simulink model "CtrlEdosObs0x2810x29"  (R2023a)
settings: Solver=ode4  StartTime=0.0  StopTime=5  FixedStep=0.001  RelTol=1e-3
values from neighbouring files (symbols this model uses):
  A = [-6 -3 -2;22 5 10;-12 0 -7]    [eje4_par3.m]    (also in ejer1_par3.m = [9 -28 -40; 10 -28 -35;-4 11 12]; ejer2_par3.m = [8 -12 4;3 -4 1;-21 30 -11]; ejer3_par3.m = [101 -6 56;-121 4 -65;-208 12 -115]; ejer5_par3.m = [-16 -25 25; -7 -12 9;-17 -26 23])
  B = [-8;11;9]    [eje4_par3.m]    (also in ejer2_par3.m = [6;-6;-32]; ejer3_par3.m = [-1;2;2]; ejer5_par3.m = [-2;0;-2])
  C = [50 20 22]    [eje4_par3.m]    (also in ejer3_par3.m = [-108 6 -58])
  k = place(A,B,lamC)    [eje4_par3.m]    (also in ejer5_par3.m = inv(R)*B'*Pk)
  L = place(A',C',lamObs')'    [eje4_par3.m]    (also in ejer3_par3.m = place(A',C',lamR')')
  Ueq1 = 3    [eje4_par3.m]    (also in ejer2_par3.m = 10)
  x0 = [3;-9;8]    [eje4_par3.m]    (also in ejer2_par3.m = [-3,9,-10]; ejer3_par3.m = [-10;-7;-7])
  x0h = [0;0;0]    [eje4_par3.m]    (also in ejer3_par3.m)
  Xeq1 = mldivide(Aeq,-Beq)    [eje4_par3.m]    (also in ejer2_par3.m)
settings Model: Creator=itzel  LastModifiedBy=userh
settings OptimizationCC: ReuseModelBlockBuffer=off

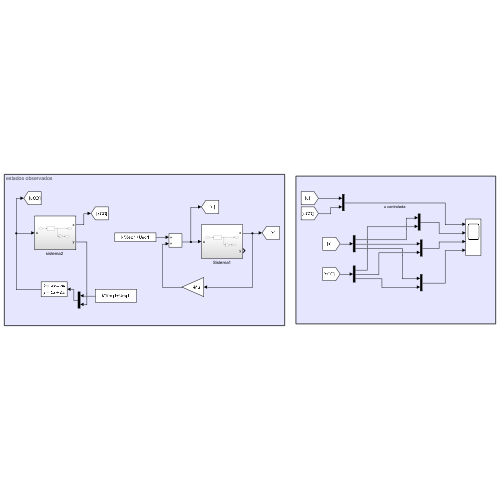
[thumbnail: Simulink's stored preview of the top-level diagram]
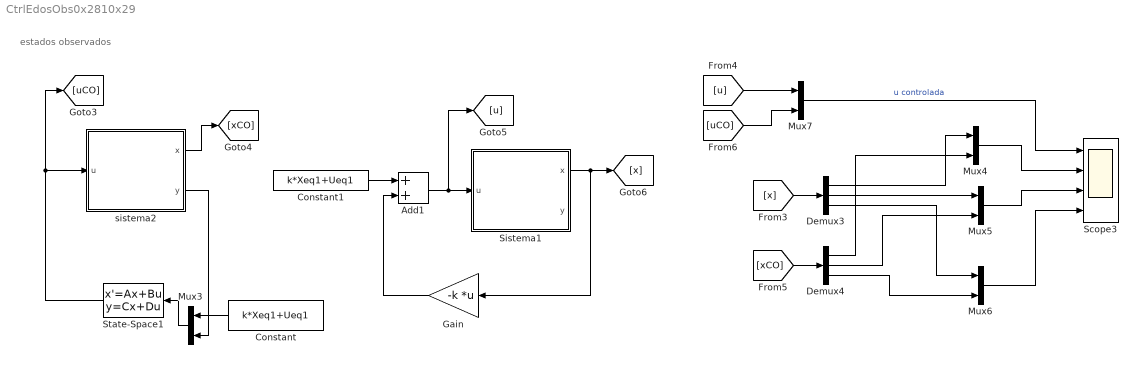
== system CtrlEdosObs0x2810x29 ==
  note: estados observados
  Add1 : Sum
  Constant : Constant  Value=k*Xeq1+Ueq1
  Constant1 : Constant  Value=k*Xeq1+Ueq1
  Demux3 : Demux  Outputs=3
  Demux4 : Demux  Outputs=3
  Gain : Gain  Gain=-k  Multiplication=Matrix(K*u)
  Mux{3..7} (5 alike) : Mux  Inputs=2
  Scope3 : Scope  NumInputPorts=4
  Sistema1 : Subsystem
  State-Space1 : StateSpace  A=A-(L*C)-(B*k)  B=[B,L]  C=-k  D=[1,0]  InitialCondition=x0h
  "sistema2 " : Subsystem
  wires:
  Constant1/1 -> Add1/1
  Sistema1/1(x) -> Gain/1, [x]
  Gain/1 -> Add1/2
  Mux7/1 -> Scope3/1  "u controlada"
  [xCO] -> Demux4/1
  Demux4/2 -> Mux5/2
  [x] -> Demux3/1
  Demux4/3 -> Mux6/2
  Demux3/3 -> Mux6/1
  Demux3/1 -> Mux4/1
  Demux3/2 -> Mux5/1
  Mux5/1 -> Scope3/3
  Mux6/1 -> Scope3/4
  Demux4/1 -> Mux4/2
  "sistema2 "/1(x) -> [xCO]
  [uCO] -> Mux7/2
  Add1/1 -> [u], Sistema1/1(u)
  Mux4/1 -> Scope3/2
  "sistema2 "/2(y) -> Mux3/2
  Constant/1 -> Mux3/1
  [u] -> Mux7/1
  State-Space1/1 -> [uCO], "sistema2 "/1(u)
  Mux3/1 -> State-Space1/1

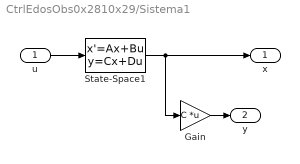
== system CtrlEdosObs0x2810x29/Sistema1 ==
  u : Inport
  Gain : Gain  Gain=C  Multiplication=Matrix(K*u)
  State-Space1 : StateSpace  A=A  B=B  C=eye(3)  D=zeros(3,1)  InitialCondition=x0  ParameterTunability=Optimized
  x : Outport
  y : Outport  Port=2
  wires:
  u/1 -> State-Space1/1
  State-Space1/1 -> Gain/1, x/1
  Gain/1 -> y/1

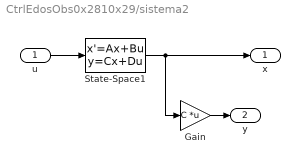
== system CtrlEdosObs0x2810x29/sistema2  ==
  u : Inport
  Gain : Gain  Gain=C  Multiplication=Matrix(K*u)
  State-Space1 : StateSpace  A=A  B=B  C=eye(3)  D=zeros(3,1)  InitialCondition=x0  ParameterTunability=Optimized
  x : Outport
  y : Outport  Port=2
  wires:
  Gain/1 -> y/1
  State-Space1/1 -> x/1, Gain/1
  u/1 -> State-Space1/1
